simulink model "CRA_Assignment1"  (R2022b)
settings: Solver=ode23  StartTime=0.0  StopTime=3600*24  RelTol=1e-7  AbsTol=1e-7
libraries: simulink x2
settings Model: Creator=lerio  LastModifiedBy=Andrea

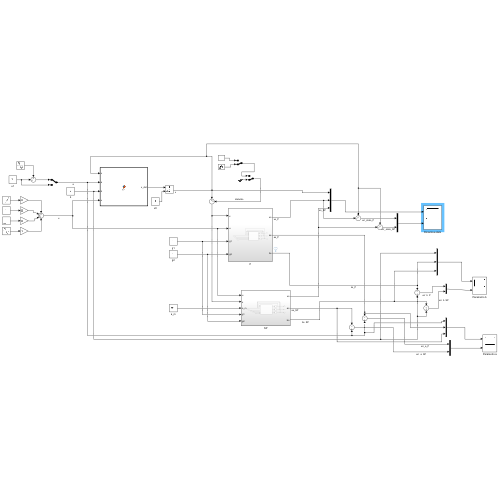
[thumbnail: Simulink's stored preview of the top-level diagram]
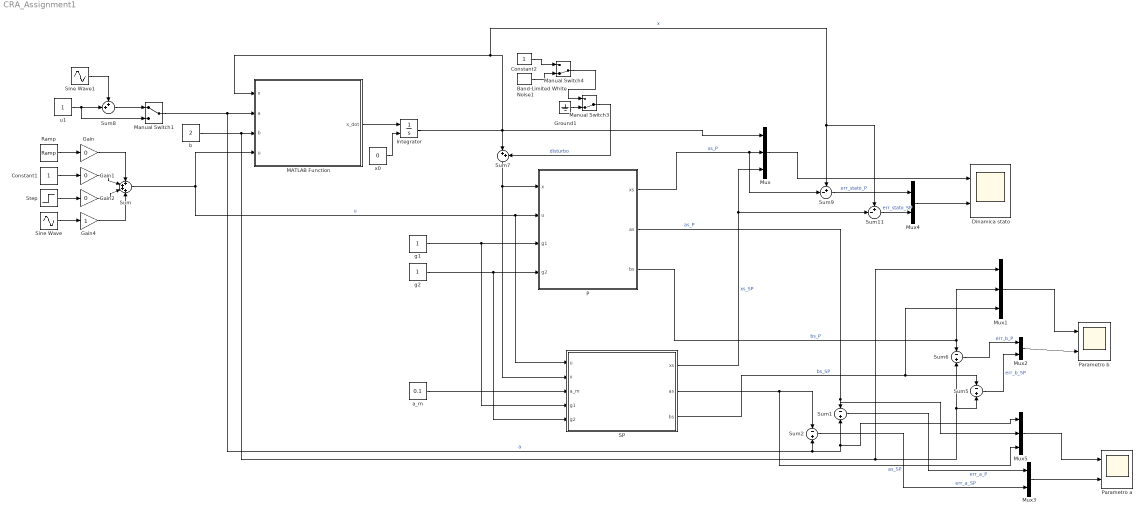
== system CRA_Assignment1 ==
  Band-Limited White Noise1 : simulink/Sources/Band-Limited White Noise  Cov=[0.1]  Ts=0.1  seed=[23341]
  Constant1 : Constant
  Constant2 : Constant
  Dinamica stato : Scope  NumInputPorts=2
  Gain : Gain  Gain=0
  Gain1 : Gain  Gain=0
  Gain2 : Gain  Gain=0
  Gain4 : Gain
  Ground1 : Ground
  Integrator : Integrator  InitialConditionSource=external
  MATLAB Function : MATLAB Function  TreatAsAtomicUnit=on
  Manual Switch1 : ManualSwitch
  Manual Switch3 : ManualSwitch  CurrentSetting=0
  Manual Switch4 : ManualSwitch  CurrentSetting=0
  Mux : Mux  Inputs=3
  Mux1 : Mux  Inputs=3
  Mux2 : Mux  Inputs=2
  Mux3 : Mux  Inputs=2
  Mux4 : Mux  Inputs=2
  Mux5 : Mux  Inputs=3
  P : Subsystem
  Parametro a : Scope  NumInputPorts=2
  Parametro b : Scope  NumInputPorts=2
  Ramp : simulink/Sources/Ramp  slope=1  start=0  InitialOutput=0
  SP : Subsystem
  Sine Wave : Sin  SampleTime=0
  Sine Wave1 : Sin  Amplitude=0.1  Frequency=(2*pi)/(24*3600)  SampleTime=0
  Step : Step  SampleTime=0
  Sum : Sum  Inputs=++++
  Sum1 : Sum  Inputs=-+
  Sum11 : Sum  Inputs=+-|
  Sum2 : Sum  Inputs=-+
  Sum5 : Sum  Inputs=-|+
  Sum6 : Sum  Inputs=-|+
  Sum7 : Sum  Inputs=|++
  Sum8 : Sum  Inputs=++|
  Sum9 : Sum  Inputs=+-|
  a_m : Constant  Value=0.1
  b : Constant  Value=2
  g1 : Constant
  g2 : Constant
  u1 : Constant
  x0 : Constant  Value=0
  wires:
  b/1 -> Mux1/1, Sum5/2, Sum6/2, MATLAB Function/3(b)
  Manual Switch1/1 -> Mux5/1, Sum1/2, Sum2/2, MATLAB Function/2(a)  "a"
  Ramp/1 -> Gain/1
  Step/1 -> Gain2/1
  Gain/1 -> Sum/1
  Gain1/1 -> Sum/2
  Gain2/1 -> Sum/3
  Sum/1 -> SP/1(u), P/2(u), MATLAB Function/4(u)  "u"
  MATLAB Function/1(x_dot) -> Integrator/1
  g1/1 -> SP/4(g1), P/3(g1)
  g2/1 -> SP/5(g2), P/4(g2)
  a_m/1 -> SP/3(a_m)
  P/1(xs) -> Sum9/2, Mux/2  "xs_P"
  SP/1(xs) -> Sum11/2, Mux/3  "xs_SP"
  P/2(as) -> Mux5/2, Sum1/1  "as_P"
  SP/2(as) -> Mux5/3, Sum2/1  "as_SP"
  Sum1/1 -> Mux3/1  "err_a_P"
  P/3(bs) -> Mux1/2, Sum6/1  "bs_P"
  SP/3(bs) -> Mux1/3, Sum5/1  "bs_SP"
  Sum6/1 -> Mux2/1  "err_b_P"
  Sum5/1 -> Mux2/2  "err_b_SP"
  Constant1/1 -> Gain1/1
  Sine Wave1/1 -> Sum8/1
  Sum8/1 -> Manual Switch1/1
  u1/1 -> Manual Switch1/2, Sum8/2
  Sine Wave/1 -> Gain4/1
  Gain4/1 -> Sum/4
  Integrator/1 -> Sum7/1, Mux/1, Sum11/1, Sum9/1, MATLAB Function/1(x)  "x"
  x0/1 -> Integrator/2
  Manual Switch4/1 -> Manual Switch3/1
  Band-Limited White Noise1/1 -> Manual Switch4/2
  Constant2/1 -> Manual Switch4/1
  Ground1/1 -> Manual Switch3/2
  Sum7/1 -> P/1(x), SP/2(x)
  Manual Switch3/1 -> Sum7/2  "disturbo"
  Mux/1 -> Dinamica stato/1
  Mux2/1 -> Parametro b/2
  Sum2/1 -> Mux3/2  "err_a_SP"
  Sum11/1 -> Mux4/2  "err_stato_SP"
  Sum9/1 -> Mux4/1  "err_stato_P"
  Mux4/1 -> Dinamica stato/2
  Mux1/1 -> Parametro b/1
  Mux5/1 -> Parametro a/1
  Mux3/1 -> Parametro a/2

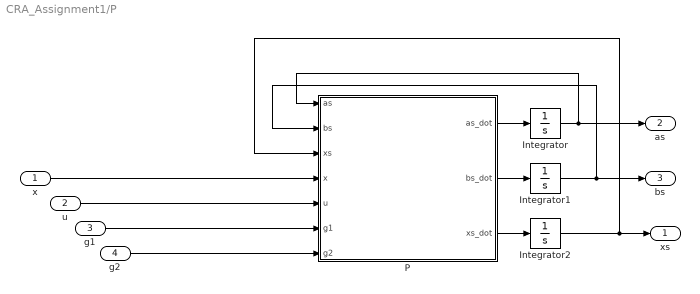
== system CRA_Assignment1/P ==
  x : Inport
  u : Inport  Port=2
  g1 : Inport  Port=3
  g2 : Inport  Port=4
  Integrator : Integrator
  Integrator1 : Integrator
  Integrator2 : Integrator
  P : MATLAB Function  TreatAsAtomicUnit=on
  xs : Outport
  as : Outport  Port=2
  bs : Outport  Port=3
  wires:
  g2/1 -> P/7(g2)
  u/1 -> P/5(u)
  g1/1 -> P/6(g1)
  x/1 -> P/4(x)
  P/1(as_dot) -> Integrator/1
  P/2(bs_dot) -> Integrator1/1
  P/3(xs_dot) -> Integrator2/1
  Integrator2/1 -> P/3(xs), xs/1
  Integrator1/1 -> P/2(bs), bs/1
  Integrator/1 -> P/1(as), as/1

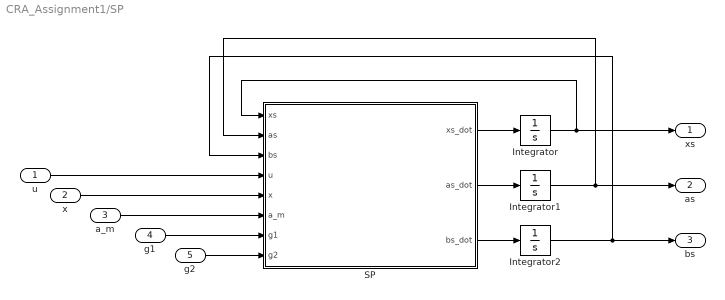
== system CRA_Assignment1/SP ==
  u : Inport
  x : Inport  Port=2
  a_m : Inport  Port=3
  g1 : Inport  Port=4
  g2 : Inport  Port=5
  Integrator : Integrator
  Integrator1 : Integrator
  Integrator2 : Integrator
  SP : MATLAB Function  TreatAsAtomicUnit=on
  xs : Outport
  as : Outport  Port=2
  bs : Outport  Port=3
  wires:
  u/1 -> SP/4(u)
  x/1 -> SP/5(x)
  g1/1 -> SP/7(g1)
  g2/1 -> SP/8(g2)
  a_m/1 -> SP/6(a_m)
  SP/1(xs_dot) -> Integrator/1
  Integrator/1 -> SP/1(xs), xs/1
  Integrator2/1 -> SP/3(bs), bs/1
  SP/3(bs_dot) -> Integrator2/1
  SP/2(as_dot) -> Integrator1/1
  Integrator1/1 -> SP/2(as), as/1

== matlab function CRA_Assignment1/P/P ==
  data: as_dot output; bs_dot output; as input; bs input; xs input; x input; u input; xs_dot output; g1 input; g2 input
function [as_dot,bs_dot,xs_dot] = fcn(as,bs,xs,x,u,g1,g2)
e = x - xs;
xs_dot = -as*xs + bs*u;
as_dot = -e*xs*g1;
bs_dot = e*u*g2;

== matlab function CRA_Assignment1/MATLAB Function ==
  data: x input; a input; b input; u input; x_dot output
function x_dot = fcn(x,a,b,u)
x_dot = -a*x+b*u;

== matlab function CRA_Assignment1/SP/SP ==
  data: xs input; as input; bs input; u input; xs_dot output; x input; a_m input; g1 input; g2 input; as_dot output; bs_dot output
function [xs_dot,as_dot,bs_dot] = fcn(xs,as,bs,u,x,a_m,g1,g2)
e = x-xs;
xs_dot = -a_m*xs+(a_m-as)*x+bs*u;
as_dot = -e*x*g1;
bs_dot = e*u;
